simulink model "Reforce_Experiment_FCS"  (R2021a)
settings: Solver=FixedStepDiscrete  StartTime=0.0  StopTime=Inf  FixedStep=Ts  RelTol=1e-3
PostLoadFcn:
  | , if any(exist('dsrtsu_mdlpostloadfcn', 'file') ~= 0), dsrtsu_mdlpostloadfcn('Execute', bdroot); end,
InitFcn:
  | , if any(exist('rtifpga_mdlclblib', 'file') ~= 0), rtifpga_mdlclblib('Init', bdroot); end,
model workspace (MAT data in the model file):
  FPGA_Control_Scheme_1_Buffer_1_1_1_write : Simulink.Signal (value not decoded)
  FPGA_Control_Scheme_1_Buffer_2_1_1_write : Simulink.Signal (value not decoded)
  FPGA_Control_Scheme_1_Register_1_1_1_write : Simulink.Signal (value not decoded)
  FPGA_Control_Scheme_1_Register_2_1_1_write : Simulink.Signal (value not decoded)
values from neighbouring files (symbols this model uses):
  abc2alphabeta0 = [      2/3      -1/3       -1/3 ... (first row only)    [Reforce_Init.m]
  alphabeta02abc = [  1          0 1/sqrt(2) ... (first row only)    [Reforce_Init.m]
  torque_ref_sample_lower = -torque_ref_sample_upper    (= -6.5)    [Reforce_Init.m]
  torque_ref_sample_upper = 6.5    [Reforce_Init.m]
  Ts = 50e-6    (= 5e-05)    [Reforce_Init.m]
undefined symbols (not defined in the file or in its folder): controller, gcbh, init_layer_0, init_layer_1, init_layer_2, init_layer_3, init_layer_4, init_layer_5, init_layer_6, init_layer_7, init_layer_8, init_layer_9, inverter, load, motor, PLL, rtimp_mpsetup_gui, sensor
libraries: simulink x14, rtiproclib x13, rti1202lib_adc_class1 x8, rti1202lib_dio_class1 x4, dspfdesign x4, rtiemclib x2, rti1202lib_dac_class1 x1, embmathops x1, rti1202lib_base x1, rtitasklib x1, dsextras x1, simulink_extras x1
(part 4 of 5)

== system Reforce_Experiment_FCS/Control_Scheme/Reconfigure_Network ==
  function : TriggerPort  TriggerType=function-call  VariantControl=(inherit)
  Constant10 : Constant  Value=10
  Constant13 : Constant  Value=90
  Default CPU Block2 : Subsystem  Commented=on  mask(Default_CPU){default_cpu=cpu2}
      mask prompts: default_cpu "Default CPU:"
      mask help: The Default CPU block defines the CPU to which separated blocks on block diagram root or in triggered subsystems are assigned.
      mask init:
      | block_revnr=200;
      mask Help: eval('rtimphelp(gcbh);');
      mask Display: disp(['Default CPU:\n ' default_cpu]);
  PROC_XDATA_WRITE_BL1 : rtiproclib/PROC_XDATA_WRITE_BL1  DSProperties=struct('RTI',struct('Version',uint32(6),'BlockType',struct('isSLSource',uint8(0),'isSLSink',uint8(1),'isHWSource',uint8(0),'isHWSink',uint8(0),'isSetup',uint8(0),'isInline',uint8(1),'isNonInline',uint8(0),'isInterrupt',uint8(0),'isChannelwise',uint8(0)),'IOBoardType','DSPROC','UnitType','','Identifier','PHSWRITE','DialogType','ML','BlockSet','DSPROC','SlaveProcessor',''))  RTIBlockInterface=struct('InputPortsActive',true,'InputPortsWidth',{{'DYNAMICALLY_SIZED'}},'InputPortsDataType',{{'SS_DOUBLE'}},'InputPortsName',{{'Data'}},'InitLevel',3,'DialogFcn','rtiprocphswritegui','BlockDisplay',{{['Register Out 1\nupdated_layer\nGroup: - Board: 1'],'auto'}},'IconTransparency','on','BlockName',struct('Token',{{'PROC_XDATA_WRITE_BL1'}}))  RTIBlockParameters=struct('BoardNo',{{'1','OFF',[1 16]}},'ChannelNo',{{'1','OFF',[]}},'AccessTyp',{{'Register','OFF',[]}},'BinaryPoint',{{'0','OFF',[]}},'DataFormat',{{'signed','OFF',[]}},'BufferLength',{{'0','OFF',[]}},'GroupNo',{{'0','OFF',[]}},'MultiChAccess',{{'0','OFF',[]}},'InitOnly',{{'0','OFF',[]}},'InitValue',{{'0','OFF',[]}},'TLCFileName',{{'rtiprocphswrite','OFF',[]}},'ModelPortBlock',{{{struct('BlockId','','SignalId','')},'OFF',[]}})  RTISFcnParameters=struct('BoardNo','double','ChannelNo','double','GroupNo','double','AccessTyp','char','BinaryPoint','double','DataFormat','char','BufferLength','double','InitOnly','double','InitValue','double','TLCFileName','char')  RTIBlockParaDefault=struct('BoardNo','1','ChannelNo','0','AccessTyp','Register','BinaryPoint','10','DataFormat','signed','BufferLength','16','GroupNo','0','MultiChAccess','0','InitOnly','0','InitValue','0','TLCFileName','rtiprocphswrite','ModelPortBlock',{{struct('BlockId','','SignalId','','BusObject','')}})
  PROC_XDATA_WRITE_BL2 : rtiproclib/PROC_XDATA_WRITE_BL1  DSProperties=struct('RTI',struct('Version',uint32(6),'BlockType',struct('isSLSource',uint8(0),'isSLSink',uint8(1),'isHWSource',uint8(0),'isHWSink',uint8(0),'isSetup',uint8(0),'isInline',uint8(1),'isNonInline',uint8(0),'isInterrupt',uint8(0),'isChannelwise',uint8(0)),'IOBoardType','DSPROC','UnitType','','Identifier','PHSWRITE','DialogType','ML','BlockSet','DSPROC','SlaveProcessor',''))  RTIBlockInterface=struct('InputPortsActive',true,'InputPortsWidth',{{'DYNAMICALLY_SIZED'}},'InputPortsDataType',{{'SS_DOUBLE'}},'InputPortsName',{{'Data'}},'InitLevel',3,'DialogFcn','rtiprocphswritegui','BlockDisplay',{{['Register Out 2\nupdated_neuron\nGroup: - Board: 1'],'auto'}},'IconTransparency','on','BlockName',struct('Token',{{'PROC_XDATA_WRITE_BL1'}}))  RTIBlockParameters=struct('BoardNo',{{'1','OFF',[1 16]}},'ChannelNo',{{'2','OFF',[]}},'AccessTyp',{{'Register','OFF',[]}},'BinaryPoint',{{'0','OFF',[]}},'DataFormat',{{'signed','OFF',[]}},'BufferLength',{{'0','OFF',[]}},'GroupNo',{{'0','OFF',[]}},'MultiChAccess',{{'0','OFF',[]}},'InitOnly',{{'0','OFF',[]}},'InitValue',{{'0','OFF',[]}},'TLCFileName',{{'rtiprocphswrite','OFF',[]}},'ModelPortBlock',{{{struct('BlockId','','SignalId','')},'OFF',[]}})  RTISFcnParameters=struct('BoardNo','double','ChannelNo','double','GroupNo','double','AccessTyp','char','BinaryPoint','double','DataFormat','char','BufferLength','double','InitOnly','double','InitValue','double','TLCFileName','char')  RTIBlockParaDefault=struct('BoardNo','1','ChannelNo','0','AccessTyp','Register','BinaryPoint','10','DataFormat','signed','BufferLength','16','GroupNo','0','MultiChAccess','0','InitOnly','0','InitValue','0','TLCFileName','rtiprocphswrite','ModelPortBlock',{{struct('BlockId','','SignalId','','BusObject','')}})
  Subsystem : Subsystem
  weight : rtiproclib/PROC_XDATA_WRITE_BL1  DSProperties=struct('RTI',struct('Version',uint32(6),'BlockType',struct('isSLSource',uint8(0),'isSLSink',uint8(1),'isHWSource',uint8(0),'isHWSink',uint8(0),'isSetup',uint8(0),'isInline',uint8(1),'isNonInline',uint8(0),'isInterrupt',uint8(0),'isChannelwise',uint8(0)),'IOBoardType','DSPROC','UnitType','','Identifier','PHSWRITE','DialogType','ML','BlockSet','DSPROC','SlaveProcessor',''))  RTIBlockInterface=struct('InputPortsActive',true,'InputPortsWidth',{{'DYNAMICALLY_SIZED'}},'InputPortsDataType',{{'SS_DOUBLE'}},'InputPortsName',{{'Data'}},'InitLevel',3,'DialogFcn','rtiprocphswritegui','BlockDisplay',{{['Buffer Out 2\nweight\nBoard: 1'],'auto'}},'IconTransparency','on','BlockName',struct('Token',{{'PROC_XDATA_WRITE_BL1'}}))  RTIBlockParameters=struct('BoardNo',{{'1','OFF',[1 16]}},'ChannelNo',{{'2','OFF',[]}},'AccessTyp',{{'Buffer','OFF',[]}},'BinaryPoint',{{'30','OFF',[]}},'DataFormat',{{'signed','OFF',[]}},'BufferLength',{{'91','OFF',[]}},'GroupNo',{{'0','OFF',[]}},'MultiChAccess',{{'0','OFF',[]}},'InitOnly',{{'0','OFF',[]}},'InitValue',{{'0','OFF',[]}},'TLCFileName',{{'rtiprocphswrite','OFF',[]}},'ModelPortBlock',{{{struct('BlockId','','SignalId','')},'OFF',[]}})  RTISFcnParameters=struct('BoardNo','double','ChannelNo','double','GroupNo','double','AccessTyp','char','BinaryPoint','double','DataFormat','char','BufferLength','double','InitOnly','double','InitValue','double','TLCFileName','char')  RTIBlockParaDefault=struct('BoardNo','1','ChannelNo','0','AccessTyp','Register','BinaryPoint','10','DataFormat','signed','BufferLength','16','GroupNo','0','MultiChAccess','0','InitOnly','0','InitValue','0','TLCFileName','rtiprocphswrite','ModelPortBlock',{{struct('BlockId','','SignalId','','BusObject','')}})
  wires:
  Subsystem/2(weights) -> weight/1
  Subsystem/1(update_layer) -> PROC_XDATA_WRITE_BL1/1
  Constant10/1 -> Subsystem/1(nb_layers)
  Subsystem/3(update_neuron) -> PROC_XDATA_WRITE_BL2/1
  Constant13/1 -> Subsystem/2(nb_neurons)

== system Reforce_Experiment_FCS/Control_Scheme/Torque_ref_sampler ==
  Add : Sum  Inputs=+-
  Add1 : Sum
  Delay : Delay  DelayLength=1  InitialConditionSource=Input port  InitialCondition=0  ExternalReset=Rising
      settings: InputPortMap=u0,r5,p4
  Divide : Product  Inputs=**
  Random Torque Sampling1 : UniformRandomNumber  Minimum=0
  Relational Operator : RelationalOperator  Operator=<=  OutDataTypeStr=boolean  RndMeth=Simplest
  T_ref_prob : Constant  Value=load.T_ref_prob  SampleTime=-1
  When to apply Random Torque : UniformRandomNumber  Minimum=0  Seed=1
  torque_sampling_lower_limit : Constant  Value=torque_ref_sample_lower  SampleTime=-1
  torque_sampling_upper_limit : Constant  Value=torque_ref_sample_upper  SampleTime=-1
  T_ref_random : Outport
  wires:
  When to apply Random Torque/1 -> Relational Operator/1
  Delay/1 -> T_ref_random/1, Delay/1
  Relational Operator/1 -> Delay/2
  T_ref_prob/1 -> Relational Operator/2
  Divide/1 -> Add1/1
  Add1/1 -> Delay/3
  Add/1 -> Divide/2
  torque_sampling_lower_limit/1 -> Add1/2, Add/2
  Random Torque Sampling1/1 -> Divide/1
  torque_sampling_upper_limit/1 -> Add/1

== system Reforce_Experiment_FCS/Control_Scheme/speed_ref_sampler ==
  Add : Sum  Inputs=+-
  Add1 : Sum
  Compare To Constant : simulink/Logic and Bit Operations/Compare To Constant  relop=>=  const=15  OutDataTypeStr=boolean
  Constant1 : Constant  Value=load.n_me_prob
  Constant2 : Constant  Value=Ts
  Delay : Delay  DelayLength=1  InitialConditionSource=Input port  InitialCondition=0  ExternalReset=Rising
      settings: InputPortMap=u0,r5,p4
  Delay1 : Delay  DelayLength=1
  Divide : Product  Inputs=**
  OR : Logic  Operator=OR  IconShape=distinctive  AllPortsSameDT=off  OutDataTypeStr=boolean
  Plus1 : Sum
  Random Speed Sampling : UniformRandomNumber  Minimum=0
  Relational Operator : RelationalOperator  Operator=<=  OutDataTypeStr=boolean  RndMeth=Simplest
  Scheduler_Clock : Delay  DelayLength=1  ExternalReset=Either
      settings: InputPortMap=u0,r5
  When to apply Random Speed : UniformRandomNumber  Minimum=0  Seed=2
  speed_sampling_lower_limit : Constant  Value=controller.DQDTC.n_lower  SampleTime=-1
  speed_sampling_upper_limit : Constant  Value=controller.DQDTC.n_upper  SampleTime=-1
  n_random : Outport
  wires:
  When to apply Random Speed/1 -> Relational Operator/1
  Delay/1 -> n_random/1, Delay/1
  Constant1/1 -> Relational Operator/2
  Random Speed Sampling/1 -> Divide/1
  speed_sampling_upper_limit/1 -> Add/1
  speed_sampling_lower_limit/1 -> Add1/2, Add/2
  Add/1 -> Divide/2
  Divide/1 -> Add1/1
  Add1/1 -> Delay/3
  OR/1 -> Delay/2, Delay1/1
  Relational Operator/1 -> OR/1
  Plus1/1 -> Scheduler_Clock/1
  Scheduler_Clock/1 -> Compare To Constant/1, Plus1/1
  Constant2/1 -> Plus1/2
  Compare To Constant/1 -> OR/2
  Delay1/1 -> Scheduler_Clock/2

== system Reforce_Experiment_FCS/Measurement/DClink_current_Calibration ==
  DC_link_current_sensor_in : Inport
  DC_link_current_gain : Gain  Gain=sensor.current.DClink.gain
  DC_link_current_offset : Constant  Value=sensor.current.DClink.offset
  Plus : Sum
  DC_link_current : Outport
  wires:
  DC_link_current_offset/1 -> Plus/2
  DC_link_current_sensor_in/1 -> DC_link_current_gain/1
  DC_link_current_gain/1 -> Plus/1
  Plus/1 -> DC_link_current/1

== system Reforce_Experiment_FCS/Measurement/DClink_voltage_Calibration ==
  DC_link_voltage_sensor_in : Inport
  Current1_gain : Gain  Gain=sensor.voltage.DClink.gain
  Current1_offset : Constant  Value=sensor.voltage.DClink.offset
  Plus : Sum
  DC_Link_voltage : Outport
  wires:
  Plus/1 -> DC_Link_voltage/1
  Current1_gain/1 -> Plus/1
  DC_link_voltage_sensor_in/1 -> Current1_gain/1
  Current1_offset/1 -> Plus/2

== system Reforce_Experiment_FCS/Measurement/PLL ==
  epsilon_el out : Inport
  Mux4 : Mux  Inputs=2
  PLL : Subsystem
  Ts : Constant  Value=Ts  OutDataTypeStr=double
  angle modulo : Subsystem
  cos : Trigonometry  Operator=cos  NumberOfDataPoints=64
  pole pair gain : Gain  Gain=1/motor.param.p
  rad/s_2_1/min : Gain  Gain=60/(2*pi)
  sin : Trigonometry  NumberOfDataPoints=64
  Omega_me : Outport
  Omega_el : Outport  Port=2
  n_me : Outport  Port=3
  wires:
  PLL/1(Omega_el) -> Omega_el/1, pole pair gain/1
  sin/1 -> Mux4/2
  Mux4/1 -> PLL/2(phi_el_cs)
  cos/1 -> Mux4/1
  Ts/1 -> PLL/1(Ts)
  angle modulo/1("angle_[-pi, pi]") -> sin/1, cos/1
  epsilon_el out/1 -> angle modulo/1(angle_rad)
  pole pair gain/1 -> Omega_me/1, rad/s_2_1/min/1
  rad/s_2_1/min/1 -> n_me/1

== system Reforce_Experiment_FCS/Measurement/Phase1_current_Calibration ==
  phase1_current_sensor_in : Inport
  Phase1_current_gain : Gain  Gain=sensor.current.ph1.gain
  Phase2_current_offset : Constant  Value=sensor.current.ph1.offset
  Plus : Sum
  phase1_current : Outport
  wires:
  Phase2_current_offset/1 -> Plus/2
  phase1_current_sensor_in/1 -> Phase1_current_gain/1
  Phase1_current_gain/1 -> Plus/1
  Plus/1 -> phase1_current/1

== system Reforce_Experiment_FCS/Measurement/Phase2_current_Calibration ==
  phase2_current_sensor_in : Inport
  Phase2_current_gain : Gain  Gain=sensor.current.ph2.gain
  Phase2_current_offset : Constant  Value=sensor.current.ph2.offset
  Plus : Sum
  phase2_current : Outport
  wires:
  Phase2_current_offset/1 -> Plus/2
  phase2_current_sensor_in/1 -> Phase2_current_gain/1
  Phase2_current_gain/1 -> Plus/1
  Plus/1 -> phase2_current/1

== system Reforce_Experiment_FCS/Measurement/Phase3_current_Calibration ==
  phase3_current_sensor_in : Inport
  Phase3_current_gain : Gain  Gain=sensor.current.ph3.gain
  Phase3_current_offset : Constant  Value=sensor.current.ph3.offset
  Plus : Sum
  phase3_current : Outport
  wires:
  Phase3_current_offset/1 -> Plus/2
  phase3_current_sensor_in/1 -> Phase3_current_gain/1
  Phase3_current_gain/1 -> Plus/1
  Plus/1 -> phase3_current/1

== system Reforce_Experiment_FCS/Measurement/abc2dq ==
  abc : Inport
  epsilon : Inport  Port=2
  Gain1 : Gain  Gain=abc2alphabeta0  Multiplication=Matrix(K*u)
  alphabeta02dq : Subsystem
  alphabeta0 : Outport
  dq : Outport  Port=2
  wires:
  epsilon/1 -> alphabeta02dq/2(epsilon)
  Gain1/1 -> alphabeta0/1, alphabeta02dq/1(alphabeta0)
  abc/1 -> Gain1/1
  alphabeta02dq/1(dq) -> dq/1

== system Reforce_Experiment_FCS/Measurement/deg2rad ==
  position_me_degree_in : Inport
  Constant : Constant  Value=360
  Constant1 : Constant  Value=sensor.angle_calibrate.bias
  Mod : Math  Operator=mod  SaturateOnIntegerOverflow=on
  Mod1 : Math  Operator=mod  SaturateOnIntegerOverflow=on
  Sum : Sum  Inputs=++|
  deg2rad : Gain  Gain=2*pi/360
  deg2rad1 : Gain  Gain=2*pi/360
  p : Gain  Gain=motor.param.p
  p1 : Gain  Gain=1/motor.param.p
  position_el_rad : Outport
  position_el_deg : Outport  Port=2
  position_me_rad : Outport  Port=3
  wires:
  deg2rad/1 -> position_el_rad/1
  position_me_degree_in/1 -> p/1
  Mod/1 -> position_el_deg/1, deg2rad/1
  Constant/1 -> Mod1/2, Mod/2
  deg2rad1/1 -> position_me_rad/1
  Constant1/1 -> Sum/1
  p/1 -> Sum/2
  Sum/1 -> Mod/1, p1/1
  Mod1/1 -> deg2rad1/1
  p1/1 -> Mod1/1

== system Reforce_Experiment_FCS/Measurement/stator_current_calculation ==
  alpha : Inport
  beta : Inport  Port=2
  Plus : Sum  Inputs=2
  Square : Math  Operator=square  SaturateOnIntegerOverflow=on
  Square Root : Sqrt  SaturateOnIntegerOverflow=on
  Square1 : Math  Operator=square  SaturateOnIntegerOverflow=on
  Stator_Current : Outport
  wires:
  Square1/1 -> Plus/2
  Square Root/1 -> Stator_Current/1
  beta/1 -> Square1/1
  alpha/1 -> Square/1
  Plus/1 -> Square Root/1
  Square/1 -> Plus/1

== system Reforce_Experiment_FCS/Multiprocessor Setup/SubSystem ==

== system Reforce_Experiment_FCS/RTI Data/RTI Data Store ==
  RTI Data Store : Subsystem  mask(RTI_DATA_STORE){}
      mask help:
      | RTI Data Store Block. This block is used by RTI to store internal model dependent data. Deleting this block will result in data loss.
      |
      | NEVER DELETE, COPY, OR MODIFY THIS BLOCK!
      mask Help:
      | RTI Data Store Block. This block is used by RTI to store internal model dependent data. Deleting this block will result in data loss.
      | 
      | NEVER DELETE, COPY, OR MODIFY THIS BLOCK!
      mask Display: text(0.5, 0.5, ' ', 'HorizontalAlignment', 'center');

== system Reforce_Experiment_FCS/Control_Scheme/DQ_DTC/Action_Processing ==
  Q_values : Inport
  a_allowed : Inport  Port=2
  epsilon_rl : Inport  Port=3
  a_current : Inport  Port=4
  EpsilonSafetyActionSelection : MATLAB Function  TreatAsAtomicUnit=on
  EpsilonSafetyActionSelection_old : MATLAB Function  Commented=on  TreatAsAtomicUnit=on
  SwitchState LUT : LookupNDDirect  InputsSelectThisObjectFromTable=Vector  Table=inverter.mapping  RemoveProtectionInput=on
  argmax : Subsystem
  s_abc : Outport
  a_policy : Outport  Port=2
  safeguard_active : Outport  Port=3
  a_aout : Outport  Port=4
  wires:
  argmax/1(argmax_Q) -> EpsilonSafetyActionSelection_old/1(argmax_Q)
  a_current/1 -> EpsilonSafetyActionSelection/3(a_current), EpsilonSafetyActionSelection_old/3(a_current)
  epsilon_rl/1 -> EpsilonSafetyActionSelection/4(epsilon), EpsilonSafetyActionSelection_old/4(epsilon)
  a_allowed/1 -> EpsilonSafetyActionSelection/2(a_allowed), EpsilonSafetyActionSelection_old/2(a_allowed)
  Q_values/1 -> EpsilonSafetyActionSelection/1(Q_values), argmax/1(Q_values)
  SwitchState LUT/1 -> s_abc/1
  EpsilonSafetyActionSelection/1(a_out) -> a_aout/1, SwitchState LUT/1
  EpsilonSafetyActionSelection/2(a_policy) -> a_policy/1
  EpsilonSafetyActionSelection/3(safeguard_active) -> safeguard_active/1

== system Reforce_Experiment_FCS/Control_Scheme/DQ_DTC/FPGA_DQN_in ==
  feature state : Inport
  Constant2 : Constant
  Mux1 : Mux  Inputs=2
  PROC_XDATA_WRITE_BL1 - input : rtiproclib/PROC_XDATA_WRITE_BL1  DSProperties=struct('RTI',struct('Version',uint32(6),'BlockType',struct('isSLSource',uint8(0),'isSLSink',uint8(1),'isHWSource',uint8(0),'isHWSink',uint8(0),'isSetup',uint8(0),'isInline',uint8(1),'isNonInline',uint8(0),'isInterrupt',uint8(0),'isChannelwise',uint8(0)),'IOBoardType','DSPROC','UnitType','','Identifier','PHSWRITE','DialogType','ML','BlockSet','DSPROC','SlaveProcessor',''))  RTIBlockInterface=struct('InputPortsActive',true,'InputPortsWidth',{{'DYNAMICALLY_SIZED'}},'InputPortsDataType',{{'SS_DOUBLE'}},'InputPortsName',{{'Data'}},'InitLevel',3,'DialogFcn','rtiprocphswritegui','BlockDisplay',{{['Buffer Out 1\nnetwork_input\nBoard: 1'],'auto'}},'IconTransparency','on','BlockName',struct('Token',{{'PROC_XDATA_WRITE_BL1'}}))  RTIBlockParameters=struct('BoardNo',{{'1','OFF',[1 16]}},'ChannelNo',{{'1','OFF',[]}},'AccessTyp',{{'Buffer','OFF',[]}},'BinaryPoint',{{'30','OFF',[]}},'DataFormat',{{'signed','OFF',[]}},'BufferLength',{{'15','OFF',[]}},'GroupNo',{{'0','OFF',[]}},'MultiChAccess',{{'0','OFF',[]}},'InitOnly',{{'0','OFF',[]}},'InitValue',{{'0','OFF',[]}},'TLCFileName',{{'rtiprocphswrite','OFF',[]}},'ModelPortBlock',{{{struct('BlockId','','SignalId','')},'OFF',[]}})  RTISFcnParameters=struct('BoardNo','double','ChannelNo','double','GroupNo','double','AccessTyp','char','BinaryPoint','double','DataFormat','char','BufferLength','double','InitOnly','double','InitValue','double','TLCFileName','char')  RTIBlockParaDefault=struct('BoardNo','1','ChannelNo','0','AccessTyp','Register','BinaryPoint','10','DataFormat','signed','BufferLength','16','GroupNo','0','MultiChAccess','0','InitOnly','0','InitValue','0','TLCFileName','rtiprocphswrite','ModelPortBlock',{{struct('BlockId','','SignalId','','BusObject','')}})
  wires:
  Mux1/1 -> PROC_XDATA_WRITE_BL1 - input/1
  Constant2/1 -> Mux1/2
  feature state/1 -> Mux1/1

== system Reforce_Experiment_FCS/Control_Scheme/DQ_DTC/FPGA_DQN_out ==
  Mux : Mux  Inputs=8
  PROC_XDATA_READ_BL1 - out1 : rtiproclib/PROC_XDATA_READ_BL1  DSProperties=struct('RTI',struct('Version',uint32(6),'BlockType',struct('isSLSource',uint8(1),'isSLSink',uint8(0),'isHWSource',uint8(0),'isHWSink',uint8(0),'isSetup',uint8(0),'isInline',uint8(1),'isNonInline',uint8(0),'isInterrupt',uint8(0),'isChannelwise',uint8(0)),'IOBoardType','DSPROC','UnitType','','Identifier','PHSREAD','DialogType','ML','BlockSet','DSPROC','SlaveProcessor',''))  RTIBlockInterface=struct('OutputPortsActive',[1 0],'OutputPortsWidth',int32([1 3]),'OutputPortsDataType',{{'SS_DOUBLE','SS_UINT32'}},'OutputPortsName',{{'Data','Status'}},'InitLevel',3,'DialogFcn','rtiprocphsreadgui','BlockDisplay',{{['Register In 1\nout0 \nGroup: 1 Board: 1'],'auto'}},'IconTransparency','on','BlockName',struct('Token',{{'PROC_XDATA_Read_BL1'}}))  RTIBlockParameters=struct('BoardNo',{{'1','OFF',[1 16]}},'ChannelNo',{{'1','OFF',[]}},'AccessTyp',{{'Register','OFF',[]}},'BinaryPoint',{{'30','OFF',[]}},'DataFormat',{{'signed','OFF',[]}},'BufferLength',{{'0','OFF',[]}},'GroupNo',{{'1','OFF',[]}},'MultiChAccess',{{'0','OFF',[]}},'TLCFileName',{{'rtiprocphsread','OFF',[]}},'ModelPortBlock',{{{struct('BlockId','','SignalId','')},'OFF',[]}})  RTISFcnParameters=struct('BoardNo','double','ChannelNo','double','GroupNo','double','AccessTyp','char','BinaryPoint','double','DataFormat','char','BufferLength','double','TLCFileName','char')  RTIBlockParaDefault=struct('BoardNo','1','ChannelNo','0','AccessTyp','Register','BinaryPoint','10','DataFormat','unsigned','BufferLength','16','GroupNo','0','MultiChAccess','0','TLCFileName','rtiprocphsread','ModelPortBlock',{{struct('BlockId','','SignalId','','BusObject','')}})
  PROC_XDATA_READ_BL1 - out2 : rtiproclib/PROC_XDATA_READ_BL1  DSProperties=struct('RTI',struct('Version',uint32(6),'BlockType',struct('isSLSource',uint8(1),'isSLSink',uint8(0),'isHWSource',uint8(0),'isHWSink',uint8(0),'isSetup',uint8(0),'isInline',uint8(1),'isNonInline',uint8(0),'isInterrupt',uint8(0),'isChannelwise',uint8(0)),'IOBoardType','DSPROC','UnitType','','Identifier','PHSREAD','DialogType','ML','BlockSet','DSPROC','SlaveProcessor',''))  RTIBlockInterface=struct('OutputPortsActive',[1 0],'OutputPortsWidth',int32([1 3]),'OutputPortsDataType',{{'SS_DOUBLE','SS_UINT32'}},'OutputPortsName',{{'Data','Status'}},'InitLevel',3,'DialogFcn','rtiprocphsreadgui','BlockDisplay',{{['Register In 2\nout1\nGroup: 1 Board: 1'],'auto'}},'IconTransparency','on','BlockName',struct('Token',{{'PROC_XDATA_Read_BL1'}}))  RTIBlockParameters=struct('BoardNo',{{'1','OFF',[1 16]}},'ChannelNo',{{'2','OFF',[]}},'AccessTyp',{{'Register','OFF',[]}},'BinaryPoint',{{'30','OFF',[]}},'DataFormat',{{'signed','OFF',[]}},'BufferLength',{{'0','OFF',[]}},'GroupNo',{{'1','OFF',[]}},'MultiChAccess',{{'0','OFF',[]}},'TLCFileName',{{'rtiprocphsread','OFF',[]}},'ModelPortBlock',{{{struct('BlockId','','SignalId','')},'OFF',[]}})  RTISFcnParameters=struct('BoardNo','double','ChannelNo','double','GroupNo','double','AccessTyp','char','BinaryPoint','double','DataFormat','char','BufferLength','double','TLCFileName','char')  RTIBlockParaDefault=struct('BoardNo','1','ChannelNo','0','AccessTyp','Register','BinaryPoint','10','DataFormat','unsigned','BufferLength','16','GroupNo','0','MultiChAccess','0','TLCFileName','rtiprocphsread','ModelPortBlock',{{struct('BlockId','','SignalId','','BusObject','')}})
  PROC_XDATA_READ_BL1 - out3 : rtiproclib/PROC_XDATA_READ_BL1  DSProperties=struct('RTI',struct('Version',uint32(6),'BlockType',struct('isSLSource',uint8(1),'isSLSink',uint8(0),'isHWSource',uint8(0),'isHWSink',uint8(0),'isSetup',uint8(0),'isInline',uint8(1),'isNonInline',uint8(0),'isInterrupt',uint8(0),'isChannelwise',uint8(0)),'IOBoardType','DSPROC','UnitType','','Identifier','PHSREAD','DialogType','ML','BlockSet','DSPROC','SlaveProcessor',''))  RTIBlockInterface=struct('OutputPortsActive',[1 0],'OutputPortsWidth',int32([1 3]),'OutputPortsDataType',{{'SS_DOUBLE','SS_UINT32'}},'OutputPortsName',{{'Data','Status'}},'InitLevel',3,'DialogFcn','rtiprocphsreadgui','BlockDisplay',{{['Register In 3\nout2\nGroup: 1 Board: 1'],'auto'}},'IconTransparency','on','BlockName',struct('Token',{{'PROC_XDATA_Read_BL1'}}))  RTIBlockParameters=struct('BoardNo',{{'1','OFF',[1 16]}},'ChannelNo',{{'3','OFF',[]}},'AccessTyp',{{'Register','OFF',[]}},'BinaryPoint',{{'30','OFF',[]}},'DataFormat',{{'signed','OFF',[]}},'BufferLength',{{'0','OFF',[]}},'GroupNo',{{'1','OFF',[]}},'MultiChAccess',{{'0','OFF',[]}},'TLCFileName',{{'rtiprocphsread','OFF',[]}},'ModelPortBlock',{{{struct('BlockId','','SignalId','')},'OFF',[]}})  RTISFcnParameters=struct('BoardNo','double','ChannelNo','double','GroupNo','double','AccessTyp','char','BinaryPoint','double','DataFormat','char','BufferLength','double','TLCFileName','char')  RTIBlockParaDefault=struct('BoardNo','1','ChannelNo','0','AccessTyp','Register','BinaryPoint','10','DataFormat','unsigned','BufferLength','16','GroupNo','0','MultiChAccess','0','TLCFileName','rtiprocphsread','ModelPortBlock',{{struct('BlockId','','SignalId','','BusObject','')}})
  PROC_XDATA_READ_BL1 - out4 : rtiproclib/PROC_XDATA_READ_BL1  DSProperties=struct('RTI',struct('Version',uint32(6),'BlockType',struct('isSLSource',uint8(1),'isSLSink',uint8(0),'isHWSource',uint8(0),'isHWSink',uint8(0),'isSetup',uint8(0),'isInline',uint8(1),'isNonInline',uint8(0),'isInterrupt',uint8(0),'isChannelwise',uint8(0)),'IOBoardType','DSPROC','UnitType','','Identifier','PHSREAD','DialogType','ML','BlockSet','DSPROC','SlaveProcessor',''))  RTIBlockInterface=struct('OutputPortsActive',[1 0],'OutputPortsWidth',int32([1 3]),'OutputPortsDataType',{{'SS_DOUBLE','SS_UINT32'}},'OutputPortsName',{{'Data','Status'}},'InitLevel',3,'DialogFcn','rtiprocphsreadgui','BlockDisplay',{{['Register In 4\nout3\nGroup: 1 Board: 1'],'auto'}},'IconTransparency','on','BlockName',struct('Token',{{'PROC_XDATA_Read_BL1'}}))  RTIBlockParameters=struct('BoardNo',{{'1','OFF',[1 16]}},'ChannelNo',{{'4','OFF',[]}},'AccessTyp',{{'Register','OFF',[]}},'BinaryPoint',{{'30','OFF',[]}},'DataFormat',{{'signed','OFF',[]}},'BufferLength',{{'0','OFF',[]}},'GroupNo',{{'1','OFF',[]}},'MultiChAccess',{{'0','OFF',[]}},'TLCFileName',{{'rtiprocphsread','OFF',[]}},'ModelPortBlock',{{{struct('BlockId','','SignalId','')},'OFF',[]}})  RTISFcnParameters=struct('BoardNo','double','ChannelNo','double','GroupNo','double','AccessTyp','char','BinaryPoint','double','DataFormat','char','BufferLength','double','TLCFileName','char')  RTIBlockParaDefault=struct('BoardNo','1','ChannelNo','0','AccessTyp','Register','BinaryPoint','10','DataFormat','unsigned','BufferLength','16','GroupNo','0','MultiChAccess','0','TLCFileName','rtiprocphsread','ModelPortBlock',{{struct('BlockId','','SignalId','','BusObject','')}})
  PROC_XDATA_READ_BL1 - out5 : rtiproclib/PROC_XDATA_READ_BL1  DSProperties=struct('RTI',struct('Version',uint32(6),'BlockType',struct('isSLSource',uint8(1),'isSLSink',uint8(0),'isHWSource',uint8(0),'isHWSink',uint8(0),'isSetup',uint8(0),'isInline',uint8(1),'isNonInline',uint8(0),'isInterrupt',uint8(0),'isChannelwise',uint8(0)),'IOBoardType','DSPROC','UnitType','','Identifier','PHSREAD','DialogType','ML','BlockSet','DSPROC','SlaveProcessor',''))  RTIBlockInterface=struct('OutputPortsActive',[1 0],'OutputPortsWidth',int32([1 3]),'OutputPortsDataType',{{'SS_DOUBLE','SS_UINT32'}},'OutputPortsName',{{'Data','Status'}},'InitLevel',3,'DialogFcn','rtiprocphsreadgui','BlockDisplay',{{['Register In 5\nout4\nGroup: 1 Board: 1'],'auto'}},'IconTransparency','on','BlockName',struct('Token',{{'PROC_XDATA_Read_BL1'}}))  RTIBlockParameters=struct('BoardNo',{{'1','OFF',[1 16]}},'ChannelNo',{{'5','OFF',[]}},'AccessTyp',{{'Register','OFF',[]}},'BinaryPoint',{{'30','OFF',[]}},'DataFormat',{{'signed','OFF',[]}},'BufferLength',{{'0','OFF',[]}},'GroupNo',{{'1','OFF',[]}},'MultiChAccess',{{'0','OFF',[]}},'TLCFileName',{{'rtiprocphsread','OFF',[]}},'ModelPortBlock',{{{struct('BlockId','','SignalId','')},'OFF',[]}})  RTISFcnParameters=struct('BoardNo','double','ChannelNo','double','GroupNo','double','AccessTyp','char','BinaryPoint','double','DataFormat','char','BufferLength','double','TLCFileName','char')  RTIBlockParaDefault=struct('BoardNo','1','ChannelNo','0','AccessTyp','Register','BinaryPoint','10','DataFormat','unsigned','BufferLength','16','GroupNo','0','MultiChAccess','0','TLCFileName','rtiprocphsread','ModelPortBlock',{{struct('BlockId','','SignalId','','BusObject','')}})
  PROC_XDATA_READ_BL1 - out6 : rtiproclib/PROC_XDATA_READ_BL1  DSProperties=struct('RTI',struct('Version',uint32(6),'BlockType',struct('isSLSource',uint8(1),'isSLSink',uint8(0),'isHWSource',uint8(0),'isHWSink',uint8(0),'isSetup',uint8(0),'isInline',uint8(1),'isNonInline',uint8(0),'isInterrupt',uint8(0),'isChannelwise',uint8(0)),'IOBoardType','DSPROC','UnitType','','Identifier','PHSREAD','DialogType','ML','BlockSet','DSPROC','SlaveProcessor',''))  RTIBlockInterface=struct('OutputPortsActive',[1 0],'OutputPortsWidth',int32([1 3]),'OutputPortsDataType',{{'SS_DOUBLE','SS_UINT32'}},'OutputPortsName',{{'Data','Status'}},'InitLevel',3,'DialogFcn','rtiprocphsreadgui','BlockDisplay',{{['Register In 6\nout5\nGroup: 1 Board: 1'],'auto'}},'IconTransparency','on','BlockName',struct('Token',{{'PROC_XDATA_Read_BL1'}}))  RTIBlockParameters=struct('BoardNo',{{'1','OFF',[1 16]}},'ChannelNo',{{'6','OFF',[]}},'AccessTyp',{{'Register','OFF',[]}},'BinaryPoint',{{'30','OFF',[]}},'DataFormat',{{'signed','OFF',[]}},'BufferLength',{{'0','OFF',[]}},'GroupNo',{{'1','OFF',[]}},'MultiChAccess',{{'0','OFF',[]}},'TLCFileName',{{'rtiprocphsread','OFF',[]}},'ModelPortBlock',{{{struct('BlockId','','SignalId','')},'OFF',[]}})  RTISFcnParameters=struct('BoardNo','double','ChannelNo','double','GroupNo','double','AccessTyp','char','BinaryPoint','double','DataFormat','char','BufferLength','double','TLCFileName','char')  RTIBlockParaDefault=struct('BoardNo','1','ChannelNo','0','AccessTyp','Register','BinaryPoint','10','DataFormat','unsigned','BufferLength','16','GroupNo','0','MultiChAccess','0','TLCFileName','rtiprocphsread','ModelPortBlock',{{struct('BlockId','','SignalId','','BusObject','')}})
  PROC_XDATA_READ_BL1 - out7 : rtiproclib/PROC_XDATA_READ_BL1  DSProperties=struct('RTI',struct('Version',uint32(6),'BlockType',struct('isSLSource',uint8(1),'isSLSink',uint8(0),'isHWSource',uint8(0),'isHWSink',uint8(0),'isSetup',uint8(0),'isInline',uint8(1),'isNonInline',uint8(0),'isInterrupt',uint8(0),'isChannelwise',uint8(0)),'IOBoardType','DSPROC','UnitType','','Identifier','PHSREAD','DialogType','ML','BlockSet','DSPROC','SlaveProcessor',''))  RTIBlockInterface=struct('OutputPortsActive',[1 0],'OutputPortsWidth',int32([1 3]),'OutputPortsDataType',{{'SS_DOUBLE','SS_UINT32'}},'OutputPortsName',{{'Data','Status'}},'InitLevel',3,'DialogFcn','rtiprocphsreadgui','BlockDisplay',{{['Register In 7\nout6\nGroup: 1 Board: 1'],'auto'}},'IconTransparency','on','BlockName',struct('Token',{{'PROC_XDATA_Read_BL1'}}))  RTIBlockParameters=struct('BoardNo',{{'1','OFF',[1 16]}},'ChannelNo',{{'7','OFF',[]}},'AccessTyp',{{'Register','OFF',[]}},'BinaryPoint',{{'30','OFF',[]}},'DataFormat',{{'signed','OFF',[]}},'BufferLength',{{'0','OFF',[]}},'GroupNo',{{'1','OFF',[]}},'MultiChAccess',{{'0','OFF',[]}},'TLCFileName',{{'rtiprocphsread','OFF',[]}},'ModelPortBlock',{{{struct('BlockId','','SignalId','')},'OFF',[]}})  RTISFcnParameters=struct('BoardNo','double','ChannelNo','double','GroupNo','double','AccessTyp','char','BinaryPoint','double','DataFormat','char','BufferLength','double','TLCFileName','char')  RTIBlockParaDefault=struct('BoardNo','1','ChannelNo','0','AccessTyp','Register','BinaryPoint','10','DataFormat','unsigned','BufferLength','16','GroupNo','0','MultiChAccess','0','TLCFileName','rtiprocphsread','ModelPortBlock',{{struct('BlockId','','SignalId','','BusObject','')}})
  PROC_XDATA_READ_BL1 - out8 : rtiproclib/PROC_XDATA_READ_BL1  DSProperties=struct('RTI',struct('Version',uint32(6),'BlockType',struct('isSLSource',uint8(1),'isSLSink',uint8(0),'isHWSource',uint8(0),'isHWSink',uint8(0),'isSetup',uint8(0),'isInline',uint8(1),'isNonInline',uint8(0),'isInterrupt',uint8(0),'isChannelwise',uint8(0)),'IOBoardType','DSPROC','UnitType','','Identifier','PHSREAD','DialogType','ML','BlockSet','DSPROC','SlaveProcessor',''))  RTIBlockInterface=struct('OutputPortsActive',[1 0],'OutputPortsWidth',int32([1 3]),'OutputPortsDataType',{{'SS_DOUBLE','SS_UINT32'}},'OutputPortsName',{{'Data','Status'}},'InitLevel',3,'DialogFcn','rtiprocphsreadgui','BlockDisplay',{{['Register In 8\nout7\nGroup: 1 Board: 1'],'auto'}},'IconTransparency','on','BlockName',struct('Token',{{'PROC_XDATA_Read_BL1'}}))  RTIBlockParameters=struct('BoardNo',{{'1','OFF',[1 16]}},'ChannelNo',{{'8','OFF',[]}},'AccessTyp',{{'Register','OFF',[]}},'BinaryPoint',{{'30','OFF',[]}},'DataFormat',{{'signed','OFF',[]}},'BufferLength',{{'0','OFF',[]}},'GroupNo',{{'1','OFF',[]}},'MultiChAccess',{{'0','OFF',[]}},'TLCFileName',{{'rtiprocphsread','OFF',[]}},'ModelPortBlock',{{{struct('BlockId','','SignalId','')},'OFF',[]}})  RTISFcnParameters=struct('BoardNo','double','ChannelNo','double','GroupNo','double','AccessTyp','char','BinaryPoint','double','DataFormat','char','BufferLength','double','TLCFileName','char')  RTIBlockParaDefault=struct('BoardNo','1','ChannelNo','0','AccessTyp','Register','BinaryPoint','10','DataFormat','unsigned','BufferLength','16','GroupNo','0','MultiChAccess','0','TLCFileName','rtiprocphsread','ModelPortBlock',{{struct('BlockId','','SignalId','','BusObject','')}})
  Q_values : Outport
  wires:
  PROC_XDATA_READ_BL1 - out5/1 -> Mux/5
  PROC_XDATA_READ_BL1 - out3/1 -> Mux/3
  PROC_XDATA_READ_BL1 - out8/1 -> Mux/8
  PROC_XDATA_READ_BL1 - out4/1 -> Mux/4
  PROC_XDATA_READ_BL1 - out6/1 -> Mux/6
  PROC_XDATA_READ_BL1 - out1/1 -> Mux/1
  PROC_XDATA_READ_BL1 - out2/1 -> Mux/2
  PROC_XDATA_READ_BL1 - out7/1 -> Mux/7
  Mux/1 -> Q_values/1

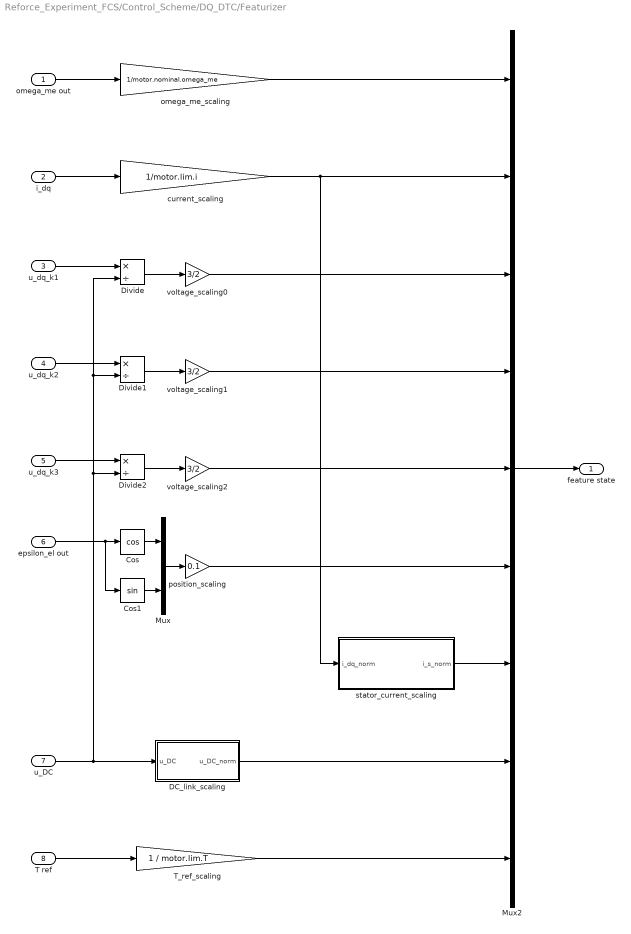
== system Reforce_Experiment_FCS/Control_Scheme/DQ_DTC/Featurizer ==
  omega_me out : Inport
  i_dq : Inport  Port=2
  u_dq_k1 : Inport  Port=3
  u_dq_k2 : Inport  Port=4
  u_dq_k3 : Inport  Port=5
  epsilon_el out : Inport  Port=6
  u_DC : Inport  Port=7
  T ref : Inport  Port=8
  Cos : Trigonometry  Operator=cos  NumberOfDataPoints=64
  Cos1 : Trigonometry  NumberOfDataPoints=64
  DC_link_scaling : Subsystem
  Divide : Product  Inputs=*/
  Divide1 : Product  Inputs=*/
  Divide2 : Product  Inputs=*/
  Mux : Mux  Inputs=2
  Mux2 : Mux  Inputs=9
  T_ref_scaling : Gain  Gain=1 / motor.lim.T
  current_scaling : Gain  Gain=1/motor.lim.i
  omega_me_scaling : Gain  Gain=1/motor.nominal.omega_me
  position_scaling : Gain  Gain=0.1
  stator_current_scaling : Subsystem
  voltage_scaling0 : Gain  Gain=3/2
  voltage_scaling1 : Gain  Gain=3/2
  voltage_scaling2 : Gain  Gain=3/2
  feature state : Outport
  wires:
  omega_me out/1 -> omega_me_scaling/1
  epsilon_el out/1 -> Cos1/1, Cos/1
  Mux/1 -> position_scaling/1
  Cos/1 -> Mux/1
  Cos1/1 -> Mux/2
  i_dq/1 -> current_scaling/1
  current_scaling/1 -> stator_current_scaling/1(i_dq_norm), Mux2/2
  omega_me_scaling/1 -> Mux2/1
  Mux2/1 -> feature state/1
  position_scaling/1 -> Mux2/6
  T ref/1 -> T_ref_scaling/1
  T_ref_scaling/1 -> Mux2/9
  voltage_scaling0/1 -> Mux2/3
  stator_current_scaling/1(i_s_norm) -> Mux2/7
  Divide/1 -> voltage_scaling0/1
  u_dq_k1/1 -> Divide/1
  u_DC/1 -> Divide2/2, Divide1/2, Divide/2, DC_link_scaling/1(u_DC)
  DC_link_scaling/1(u_DC_norm) -> Mux2/8
  Divide1/1 -> voltage_scaling1/1
  Divide2/1 -> voltage_scaling2/1
  voltage_scaling2/1 -> Mux2/5
  voltage_scaling1/1 -> Mux2/4
  u_dq_k2/1 -> Divide1/1
  u_dq_k3/1 -> Divide2/1

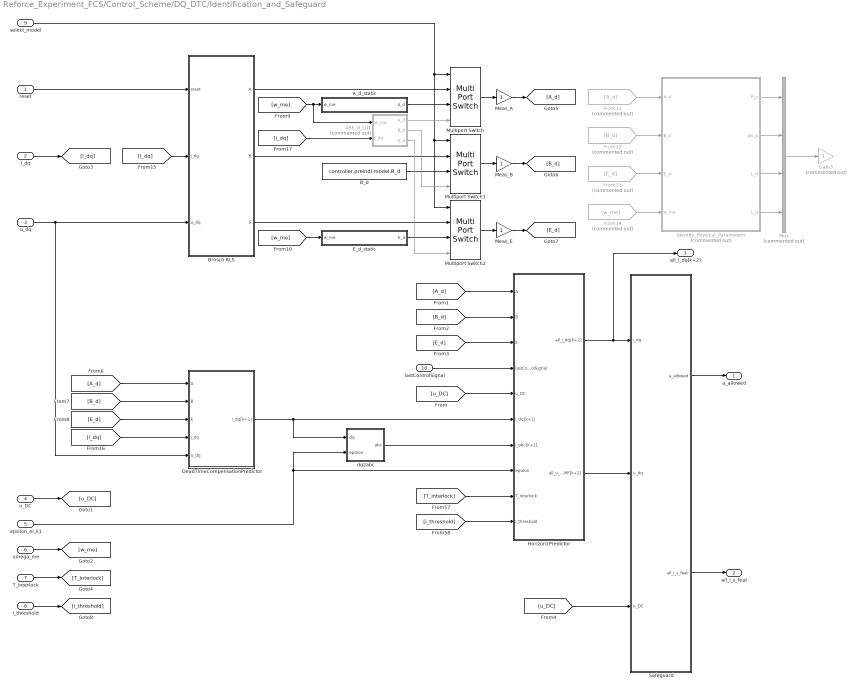
== system Reforce_Experiment_FCS/Control_Scheme/DQ_DTC/Identification_and_Safeguard ==
  reset : Inport
  i_dq : Inport  Port=2
  u_dq : Inport  Port=3
  u_DC : Inport  Port=4
  epsilon_el_k1 : Inport  Port=5
  omega_me : Inport  Port=6
  T_interlock : Inport  Port=7
  i_threshold : Inport  Port=8
  select_model : Inport  Port=9
  lastControlSignal : Inport  Port=10
  ABE_d_LUT : MATLAB Function  Commented=on  TreatAsAtomicUnit=on
  A_d_static : Subsystem
  B_d : Constant  Value=controller.preindl.model.B_d
  Brosch RLS : Subsystem
  DeadTimeCompensationPredictor : Subsystem
  E_d_static : Subsystem
  From11 : From  Commented=on  GotoTag=A_d
  From12 : From  Commented=on  GotoTag=B_d
  From13 : From  Commented=on  GotoTag=E_d
  From14 : From  Commented=on  GotoTag=w_me
  Gain3 : Gain  Commented=on
  Horizon1Predictor : Subsystem
  Identify_Physical_Parameters : Subsystem  Commented=on
  Meas_A : Gain
  Meas_B : Gain
  Meas_E : Gain
  Multiport Switch : MultiPortSwitch
  Multiport Switch1 : MultiPortSwitch
  Multiport Switch2 : MultiPortSwitch
  Mux : Mux  Commented=on
  Safeguard : Subsystem
  dq2abc : Subsystem
  a_allowed : Outport
  all_i_s_feat : Outport  Port=2
  all_i_dq[k+2] : Outport  Port=3
  wires:
  Horizon1Predictor/1(all_i_dq[k+2]) -> all_i_dq[k+2]/1, Safeguard/1(i_dq)
  [A_d] -> DeadTimeCompensationPredictor/1(A)
  [B_d] -> DeadTimeCompensationPredictor/2(B)
  [E_d] -> DeadTimeCompensationPredictor/3(E)
  Horizon1Predictor/2(all_u_EMF[k+2]) -> Safeguard/2(u_dq)
  DeadTimeCompensationPredictor/1(i_dq[k+1]) -> dq2abc/1(dq), Horizon1Predictor/6(i_dq[k+1])
  Safeguard/1(a_allowed) -> a_allowed/1
  Safeguard/2(all_i_s_feat) -> all_i_s_feat/1
  epsilon_el_k1/1 -> dq2abc/2(epsilon), Horizon1Predictor/8(epsilon)
  u_dq/1 -> Brosch RLS/3(u_dq), DeadTimeCompensationPredictor/5(u_dq)
  u_DC/1 -> [u_DC]
  [A_d] -> Horizon1Predictor/1(A)
  [E_d] -> Horizon1Predictor/3(E)
  [B_d] -> Horizon1Predictor/2(B)
  [u_DC] -> Horizon1Predictor/5(u_DC)
  [u_DC] -> Safeguard/3(u_DC)
  omega_me/1 -> [w_me]
  Multiport Switch/1 -> Meas_A/1
  Multiport Switch2/1 -> Meas_E/1
  Multiport Switch1/1 -> Meas_B/1
  Brosch RLS/3(E) -> Multiport Switch2/2
  Brosch RLS/2(B) -> Multiport Switch1/2
  Brosch RLS/1(A) -> Multiport Switch/2
  select_model/1 -> Multiport Switch2/1, Multiport Switch1/1, Multiport Switch/1
  B_d/1 -> Multiport Switch1/3
  A_d_static/1(A_d) -> Multiport Switch/3
  [w_me] -> ABE_d_LUT/1(w_me), A_d_static/1(w_me)
  [w_me] -> E_d_static/1(w_me)
  E_d_static/1(E_d) -> Multiport Switch2/3
  reset/1 -> Brosch RLS/1(reset)
  From12/1 -> Identify_Physical_Parameters/2(B_d)
  From13/1 -> Identify_Physical_Parameters/3(E_d)
  From14/1 -> Identify_Physical_Parameters/4(w_me)
  Identify_Physical_Parameters/4(L_q) -> Mux/4
  Identify_Physical_Parameters/3(L_d) -> Mux/3
  Identify_Physical_Parameters/2(psi_p) -> Mux/2
  Identify_Physical_Parameters/1(R_s) -> Mux/1
  Meas_A/1 -> [A_d]
  Meas_B/1 -> [B_d]
  Meas_E/1 -> [E_d]
  From11/1 -> Identify_Physical_Parameters/1(A_d)
  ABE_d_LUT/1(A_d) -> Multiport Switch/4
  i_dq/1 -> [i_dq]
  [i_dq] -> Brosch RLS/2(i_dq)
  [i_dq] -> DeadTimeCompensationPredictor/4(i_dq)
  [i_dq] -> ABE_d_LUT/2(i_dq)
  ABE_d_LUT/2(B_d) -> Multiport Switch1/4
  ABE_d_LUT/3(E_d) -> Multiport Switch2/4
  [T_interlock] -> Horizon1Predictor/9(T_interlock)
  [i_threshold] -> Horizon1Predictor/10(i_threshold)
  T_interlock/1 -> [T_interlock]
  i_threshold/1 -> [i_threshold]
  dq2abc/1(abc) -> Horizon1Predictor/7(i_abc[k+1])
  Mux/1 -> Gain3/1
  lastControlSignal/1 -> Horizon1Predictor/4(lastControlSignal)

== system Reforce_Experiment_FCS/Control_Scheme/DQ_DTC/Normierung der Spannungen für PWM-Register von 0 bis 1 ==
  s_abc : Inport
  Add2 : Sum
  Constant8 : Constant  Value=0.5  OutDataTypeStr=single  SampleTime=-1
  Multiply : Gain  Gain=0.5
  d_abc : Outport
  wires:
  Multiply/1 -> Add2/2
  Constant8/1 -> Add2/1
  Add2/1 -> d_abc/1
  s_abc/1 -> Multiply/1

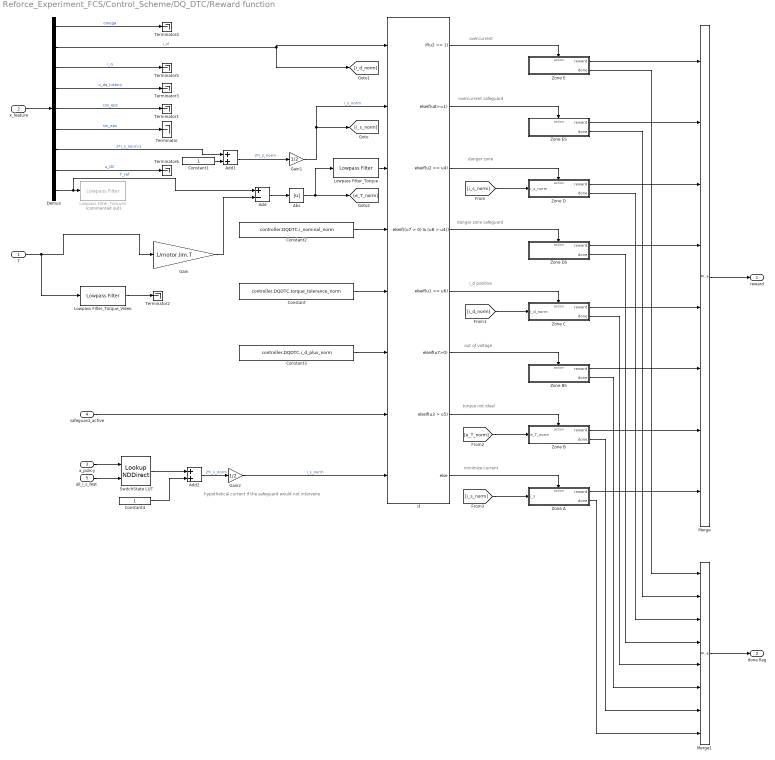
== system Reforce_Experiment_FCS/Control_Scheme/DQ_DTC/Reward function ==
  note: hypothetical current if the safeguard would not intervene
  note: minimize current
  note: torque not ideal
  note: i_d positive
  note: danger zone safeguard
  note: danger zone
  note: overcurrent
  note: overcurrent safeguard
  note: out of voltage
  T : Inport
  x_feature : Inport  Port=2
  a_policy : Inport  Port=3
  safeguard_active : Inport  Port=4
  all_i_s_feat : Inport  Port=5
  Abs : Abs
  Add : Sum  Inputs=+-
  Add1 : Sum
  Add2 : Sum
  Constant : Constant  Value=controller.DQDTC.torque_tolerance_norm
  Constant1 : Constant
  Constant2 : Constant  Value=controller.DQDTC.i_nominal_norm
  Constant3 : Constant  Value=controller.DQDTC.i_d_plus_norm
  Constant4 : Constant
  Demux : Demux  Outputs=[1 1 1 6 1 1 1 1 1]
  Gain : Gain  Gain=1/motor.lim.T
  Gain1 : Gain  Gain=1/2
  Gain2 : Gain  Gain=1/2
  If : If  NumInputs=8  IfExpression=u2 >= 1  ElseIfExpressions=u8>=1,u2 >= u4, (u7 > 0) & (u8 > u4), u1 >= u6, u7>0, u3 > u5
  Lowpass Filter_Torque : dspfdesign/Lowpass Filter  FilterType=IIR  DesignForMinimumOrder=on  FilterOrder=50  PassbandFrequency=controller.DQDTC.LP_filter.passband_edge  StopbandFrequency=controller.DQDTC.LP_filter.stopband_edge  PassbandRipple=0.1  StopbandAttenuation=80  InheritSampleRate=off  SampleRate=1/Ts  SimulateUsing=Interpreted execution  roundingMode=Floor  coeffsDataTypeStr=fixdt(1,16)
  Lowpass Filter_Torque1 : dspfdesign/Lowpass Filter  Commented=on  FilterType=IIR  DesignForMinimumOrder=on  FilterOrder=50  PassbandFrequency=controller.DQDTC.LP_filter.passband_edge  StopbandFrequency=controller.DQDTC.LP_filter.stopband_edge  PassbandRipple=0.1  StopbandAttenuation=80  InheritSampleRate=off  SampleRate=1/Ts  SimulateUsing=Interpreted execution  roundingMode=Floor  coeffsDataTypeStr=fixdt(1,16)
  Lowpass Filter_Torque_Video : dspfdesign/Lowpass Filter  FilterType=IIR  DesignForMinimumOrder=on  FilterOrder=50  PassbandFrequency=6.6  StopbandFrequency=controller.DQDTC.LP_filter.stopband_edge  PassbandRipple=0.1  StopbandAttenuation=80  InheritSampleRate=off  SampleRate=1/Ts  SimulateUsing=Interpreted execution  roundingMode=Floor  coeffsDataTypeStr=fixdt(1,16)
  Merge : Merge  Inputs=8
  Merge1 : Merge  Inputs=8
  SwitchState LUT : LookupNDDirect  NumberOfTableDimensions=1  TableIsInput=on  Table=inverter.mapping  RemoveProtectionInput=on
  Terminator{,1..6} (7 alike) : Terminator
  Zone A : Subsystem  TreatAsAtomicUnit=on
  Zone B : Subsystem  TreatAsAtomicUnit=on
  Zone BS : Subsystem  TreatAsAtomicUnit=on
  Zone C : Subsystem  TreatAsAtomicUnit=on
  Zone D : Subsystem  TreatAsAtomicUnit=on
  Zone DS : Subsystem  TreatAsAtomicUnit=on
  Zone E : Subsystem  TreatAsAtomicUnit=on
  Zone ES : Subsystem  TreatAsAtomicUnit=on
  reward : Outport
  done flag : Outport  Port=2
  wires:
  x_feature/1 -> Demux/1
  Demux/1 -> Terminator4/1  "omega"
  Demux/2 -> [i_d_norm], If/1  "i_d"
  Demux/3 -> Terminator5/1  "i_q"
  Demux/4 -> Terminator3/1  "u_dq_history"
  Demux/5 -> Terminator1/1  "cos_eps"
  Demux/6 -> Terminator/1  "sin_eps"
  Add/1 -> Abs/1
  Abs/1 -> [e_T_norm], Lowpass Filter_Torque/1
  Constant/1 -> If/5
  Constant2/1 -> If/4
  Zone E/1(reward) -> Merge/1
  Constant3/1 -> If/6
  [i_s_norm] -> Zone D/1(i_s_norm)
  [i_d_norm] -> Zone C/1(i_d_norm)
  [e_T_norm] -> Zone B/1(e_T_norm)
  [i_s_norm] -> Zone A/1(i_s)
  Demux/7 -> Add1/1  "2*i_s_norm-1"
  Constant1/1 -> Add1/2
  Add1/1 -> Gain1/1  "2*i_s_norm"
  Gain1/1 -> If/2, [i_s_norm]  "i_s_norm"
  all_i_s_feat/1 -> SwitchState LUT/2
  a_policy/1 -> SwitchState LUT/1
  SwitchState LUT/1 -> Add2/1
  Constant4/1 -> Add2/2
  Add2/1 -> Gain2/1  "2*i_s_norm"
  Gain2/1 -> If/8  "i_s_norm"
  safeguard_active/1 -> If/7
  If/1 -> Zone E/Action
  If/8 -> Zone A/Action
  If/5 -> Zone C/Action
  If/4 -> Zone DS/Action
  If/3 -> Zone D/Action
  If/2 -> Zone ES/Action
  Zone ES/1(reward) -> Merge/2
  Zone D/1(reward) -> Merge/3
  Zone DS/1(reward) -> Merge/4
  Zone C/1(reward) -> Merge/5
  If/7 -> Zone B/Action
  Zone A/1(reward) -> Merge/8
  Zone B/1(reward) -> Merge/7
  If/6 -> Zone BS/Action
  Zone BS/1(reward) -> Merge/6
  Zone A/2(done) -> Merge1/8
  Zone B/2(done) -> Merge1/7
  Zone BS/2(done) -> Merge1/6
  Zone C/2(done) -> Merge1/5
  Zone DS/2(done) -> Merge1/4
  Zone D/2(done) -> Merge1/3
  Zone ES/2(done) -> Merge1/2
  Zone E/2(done) -> Merge1/1
  Demux/8 -> Terminator6/1  "u_DC"
  Gain/1 -> Add/2
  Merge/1 -> reward/1
  Merge1/1 -> done flag/1
  Demux/9 -> Add/1, Lowpass Filter_Torque1/1  "T_ref"
  T/1 -> Lowpass Filter_Torque_Video/1, Gain/1
  Lowpass Filter_Torque_Video/1 -> Terminator2/1
  Lowpass Filter_Torque/1 -> If/3

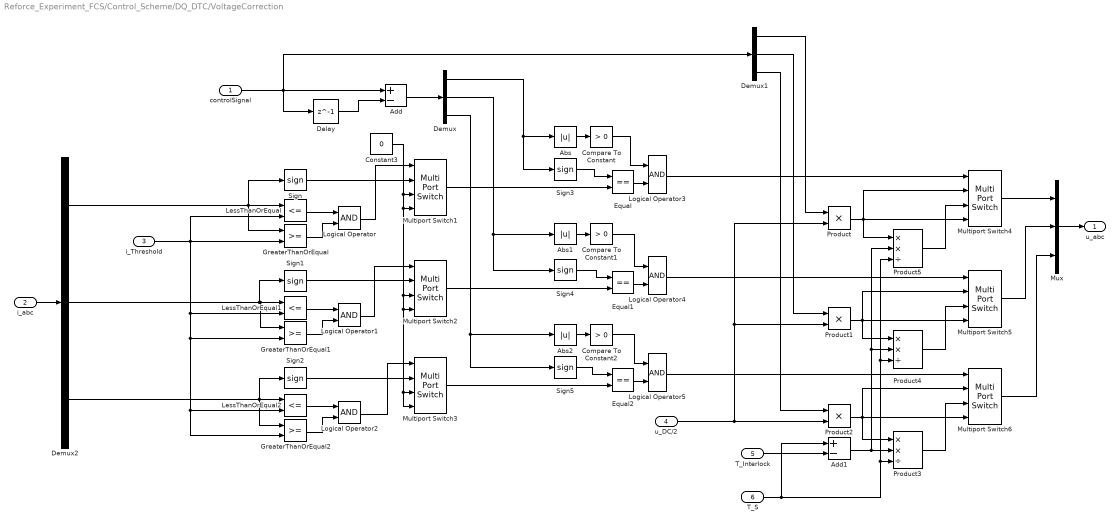
== system Reforce_Experiment_FCS/Control_Scheme/DQ_DTC/VoltageCorrection ==
  controlSignal : Inport
  i_abc : Inport  Port=2
  i_Threshold : Inport  Port=3
  u_DC/2 : Inport  Port=4
  T_Interlock : Inport  Port=5
  T_S : Inport  Port=6
  Abs : Abs
  Abs1 : Abs
  Abs2 : Abs
  Add : Sum  Inputs=+-
  Add1 : Sum  Inputs=+-
  Compare To Constant : simulink/Logic and Bit Operations/Compare To Constant  relop=>  const=0  OutDataTypeStr=boolean
  Compare To Constant1 : simulink/Logic and Bit Operations/Compare To Constant  relop=>  const=0  OutDataTypeStr=boolean
  Compare To Constant2 : simulink/Logic and Bit Operations/Compare To Constant  relop=>  const=0  OutDataTypeStr=boolean
  Constant3 : Constant  Value=0
  Delay : Delay  DelayLength=1  InitialCondition=0
  Demux : Demux  Outputs=3
  Demux1 : Demux  Outputs=3
  Demux2 : Demux  Outputs=3
  Equal : RelationalOperator  Operator===  OutDataTypeStr=boolean  RndMeth=Simplest
  Equal1 : RelationalOperator  Operator===  OutDataTypeStr=boolean  RndMeth=Simplest
  Equal2 : RelationalOperator  Operator===  OutDataTypeStr=boolean  RndMeth=Simplest
  GreaterThanOrEqual : RelationalOperator  OutDataTypeStr=boolean  RndMeth=Simplest
  GreaterThanOrEqual1 : RelationalOperator  OutDataTypeStr=boolean  RndMeth=Simplest
  GreaterThanOrEqual2 : RelationalOperator  OutDataTypeStr=boolean  RndMeth=Simplest
  LessThanOrEqual : RelationalOperator  Operator=<=  OutDataTypeStr=boolean  RndMeth=Simplest
  LessThanOrEqual1 : RelationalOperator  Operator=<=  OutDataTypeStr=boolean  RndMeth=Simplest
  LessThanOrEqual2 : RelationalOperator  Operator=<=  OutDataTypeStr=boolean  RndMeth=Simplest
  Logical Operator{,1..5} (6 alike) : Logic  AllPortsSameDT=off  OutDataTypeStr=boolean
  Multiport Switch{1..6} (6 alike) : MultiPortSwitch  DataPortOrder=Specify indices  DataPortIndices={0,1}  DataPortForDefault=Additional data port
  Mux : Mux  Inputs=3
  Product : Product
  Product1 : Product
  Product2 : Product
  Product3 : Product  Inputs=**/
  Product4 : Product  Inputs=**/
  Product5 : Product  Inputs=**/
  Sign{,1..5} (6 alike) : Signum
  u_abc : Outport
  wires:
  GreaterThanOrEqual2/1 -> Logical Operator2/2
  Constant3/1 -> Multiport Switch3/4, Multiport Switch3/3, Multiport Switch2/4, Multiport Switch2/3, Multiport Switch1/4, Multiport Switch1/3
  Demux2/1 -> GreaterThanOrEqual/1, Sign/1, LessThanOrEqual/1
  u_DC/2/1 -> Product/2, Product1/2, Product2/2
  T_S/1 -> Product5/3, Product4/3, Product3/3, Add1/1
  Demux/1 -> Sign3/1, Abs/1
  GreaterThanOrEqual1/1 -> Logical Operator1/2
  LessThanOrEqual/1 -> Logical Operator/1
  Add/1 -> Demux/1
  LessThanOrEqual1/1 -> Logical Operator1/1
  Abs2/1 -> Compare To Constant2/1
  Abs/1 -> Compare To Constant/1
  i_Threshold/1 -> LessThanOrEqual/2, GreaterThanOrEqual2/2, LessThanOrEqual2/2, GreaterThanOrEqual1/2, LessThanOrEqual1/2, GreaterThanOrEqual/2
  Product/1 -> Product5/1, Multiport Switch4/4, Multiport Switch4/2
  Add1/1 -> Product4/2, Product5/2, Product3/2
  Abs1/1 -> Compare To Constant1/1
  Multiport Switch6/1 -> Mux/3
  Demux1/2 -> Product1/1
  Multiport Switch1/1 -> Equal/2
  Multiport Switch5/1 -> Mux/2
  Product4/1 -> Multiport Switch5/3
  T_Interlock/1 -> Add1/2
  Logical Operator1/1 -> Multiport Switch2/1
  Logical Operator/1 -> Multiport Switch1/1
  GreaterThanOrEqual/1 -> Logical Operator/2
  controlSignal/1 -> Delay/1, Demux1/1, Add/1
  Compare To Constant1/1 -> Logical Operator4/1
  Demux1/1 -> Product/1
  Demux1/3 -> Product2/1
  Logical Operator4/1 -> Multiport Switch5/1
  Product5/1 -> Multiport Switch4/3
  Product1/1 -> Product4/1, Multiport Switch5/4, Multiport Switch5/2
  Logical Operator2/1 -> Multiport Switch3/1
  Delay/1 -> Add/2
  Compare To Constant/1 -> Logical Operator3/1
  Product2/1 -> Product3/1, Multiport Switch6/4, Multiport Switch6/2
  LessThanOrEqual2/1 -> Logical Operator2/1
  Sign/1 -> Multiport Switch1/2
  Product3/1 -> Multiport Switch6/3
  Logical Operator3/1 -> Multiport Switch4/1
  Sign1/1 -> Multiport Switch2/2
  Sign2/1 -> Multiport Switch3/2
  Logical Operator5/1 -> Multiport Switch6/1
  Compare To Constant2/1 -> Logical Operator5/1
  Multiport Switch4/1 -> Mux/1
  Demux2/2 -> Sign1/1, GreaterThanOrEqual1/1, LessThanOrEqual1/1
  Demux2/3 -> Sign2/1, GreaterThanOrEqual2/1, LessThanOrEqual2/1
  Equal/1 -> Logical Operator3/2
  Sign3/1 -> Equal/1
  Sign4/1 -> Equal1/1
  Multiport Switch2/1 -> Equal1/2
  Demux/2 -> Abs1/1, Sign4/1
  Equal1/1 -> Logical Operator4/2
  Demux/3 -> Sign5/1, Abs2/1
  Multiport Switch3/1 -> Equal2/2
  Sign5/1 -> Equal2/1
  Equal2/1 -> Logical Operator5/2
  Mux/1 -> u_abc/1
  i_abc/1 -> Demux2/1

== system Reforce_Experiment_FCS/Control_Scheme/DQ_DTC/abc2dq1 ==
  abc : Inport
  epsilon : Inport  Port=2
  Gain1 : Gain  Gain=abc2alphabeta0  Multiplication=Matrix(K*u)
  alphabeta02dq : Subsystem
  dq : Outport
  wires:
  alphabeta02dq/1(dq) -> dq/1
  abc/1 -> Gain1/1
  Gain1/1 -> alphabeta02dq/1(alphabeta0)
  epsilon/1 -> alphabeta02dq/2(epsilon)

== system Reforce_Experiment_FCS/Control_Scheme/Reconfigure_Network/Default CPU Block2 ==
